simulink model "gauss"  (R2022b)
settings: Solver=VariableStepAuto  StartTime=0.0  StopTime=10.0  RelTol=1e-3
libraries: commdigbbndpm3 x3, commsink2 x1, phaseddetectlib x1, commrandsrc3 x1
settings Model: Creator=Leoni Gabriel  LastModifiedBy=Leoni Gabriel

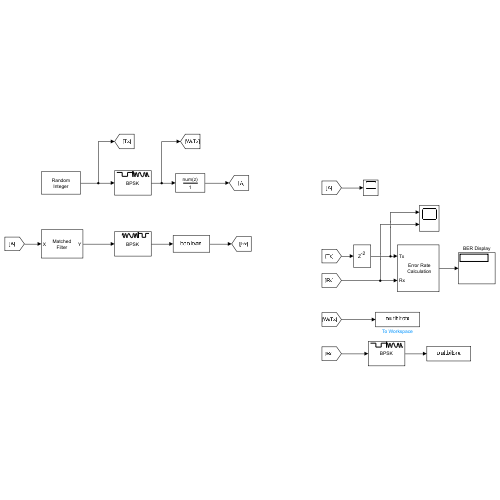
[thumbnail: Simulink's stored preview of the top-level diagram]
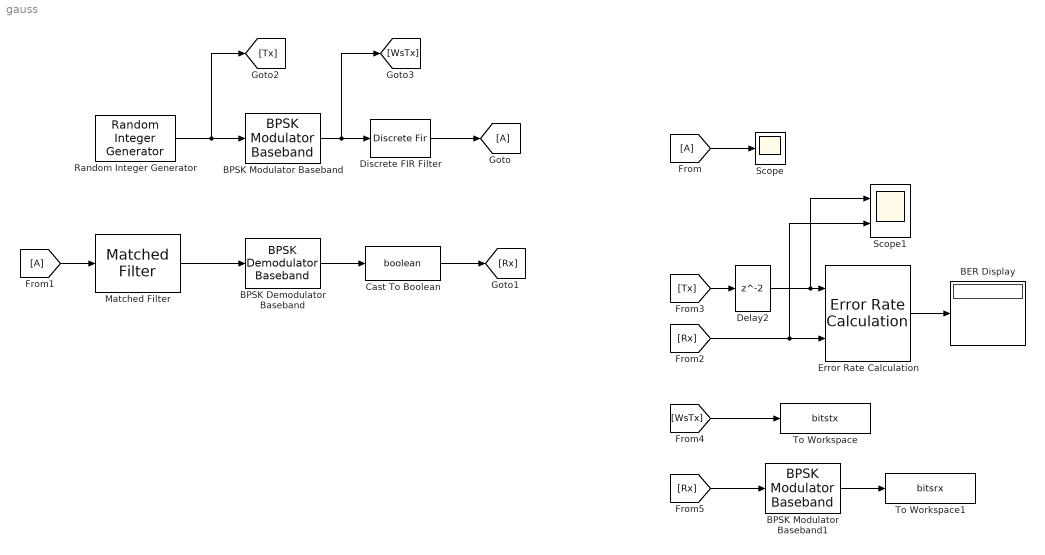
== system gauss ==
  BER Display : Display
  BPSK Demodulator Baseband : commdigbbndpm3/BPSK Demodulator Baseband  DecType=Hard decision  VarSource=Dialog  Variance=1  Ph=0  outDtype=boolean  derotateFactorWordLen=16  derotateFactorDataTypeStr=Inherit: Same word length as input  derotateFactorLastDataTypeStr=Inherit: Same word length as input
  BPSK Modulator Baseband : commdigbbndpm3/BPSK Modulator Baseband  Ph=0  outDtype=double  outWordLen=16  outUDDataType=sfix(16)  outFracLenMode=Best precision  outFracLen=15  outDataTypeStr=double  outLastDataTypeStr=double
  BPSK Modulator Baseband1 : commdigbbndpm3/BPSK Modulator Baseband  Ph=0  outDtype=double  outWordLen=16  outUDDataType=sfix(16)  outFracLenMode=Best precision  outFracLen=15  outDataTypeStr=double  outLastDataTypeStr=double
  Cast To Boolean : DataTypeConversion  OutDataTypeStr=boolean  SaturateOnIntegerOverflow=off  RndMeth=Floor
  Delay2 : Delay  UseCircularBuffer=on
  Discrete FIR Filter : DiscreteFir  Coefficients="[0.0668    0.8664    0.0668]"
  Error Rate Calculation : commsink2/Error Rate Calculation  N=0  st_delay=0  cp_mode=Entire frame  subframe=[]  PMode=Port  WsName=ErrorVec  RsMode2=off  stop=off  numErr=100  maxBits=1e6
  From : From
  From1 : From
  Goto : Goto
  Matched Filter : phaseddetectlib/Matched Filter  CoefficientsSource=Property  Coefficients="[0.0668    0.8664    0.0668]"  SpectrumWindow=None  CustomSpectrumWindow=@hamming  SpectrumRange=[ 0, 1e5 ]  SampleRateFromInputCheckbox=on  SampleRate=1e6  SidelobeAttenuation=30  Beta=0.5  Nbar=4  GainOutputPort=off  MaximumNumInputSamplesSource=Auto  MaximumNumInputSamples=100  SimulateUsing=Interpreted execution
  Random Integer Generator : commrandsrc3/Random Integer Generator  SetSize=2  SeedSource=Auto  Seed=0  SampleTime=0.001  SamplesPerFrame=1  OutputDataType=boolean  SimulateUsing=Interpreted execution
  Scope : Scope
  Scope1 : Scope  NumInputPorts=2
  To Workspace : ToWorkspace  VariableName=bitstx  SaveFormat=Timeseries  SampleTime=-1
  To Workspace1 : ToWorkspace  VariableName=bitsrx  SaveFormat=Timeseries  SampleTime=-1
  wires:
  Error Rate Calculation/1 -> BER Display/1
  Delay2/1 -> Scope1/1, Error Rate Calculation/1
  Random Integer Generator/1 -> [Tx], BPSK Modulator Baseband/1
  BPSK Modulator Baseband/1 -> [WsTx], Discrete FIR Filter/1
  Discrete FIR Filter/1 -> Goto/1
  From1/1 -> Matched Filter/1
  Matched Filter/1 -> BPSK Demodulator Baseband/1
  BPSK Demodulator Baseband/1 -> Cast To Boolean/1
  Cast To Boolean/1 -> [Rx]
  From/1 -> Scope/1
  [Tx] -> Delay2/1
  [Rx] -> Error Rate Calculation/2, Scope1/2
  [WsTx] -> To Workspace/1
  BPSK Modulator Baseband1/1 -> To Workspace1/1
  [Rx] -> BPSK Modulator Baseband1/1
